simulink model "daohang_2017b"  (R2017b)
settings: Solver=FixedStepAuto  StartTime=0.0  StopTime=80  FixedStep=0.01  MaxStep=0.01  RelTol=1e-3
undefined symbols (not defined in the file or in its folder): Earth, ini, Newton, Raphson, WGS84
libraries: sharedutil x2, sharedtransform x2, simulink_extras x2, shared6dof x1, aerolibatmos2 x1, aerolibobsolete x1, aerolibtransform2 x1
(part 1 of 2)
settings Model: Creator=d8230  LastModifiedBy=d8230
settings SFSimCC: SimUseLocalCustomCode=on
settings RTWCC: RTWUseLocalCustomCode=on

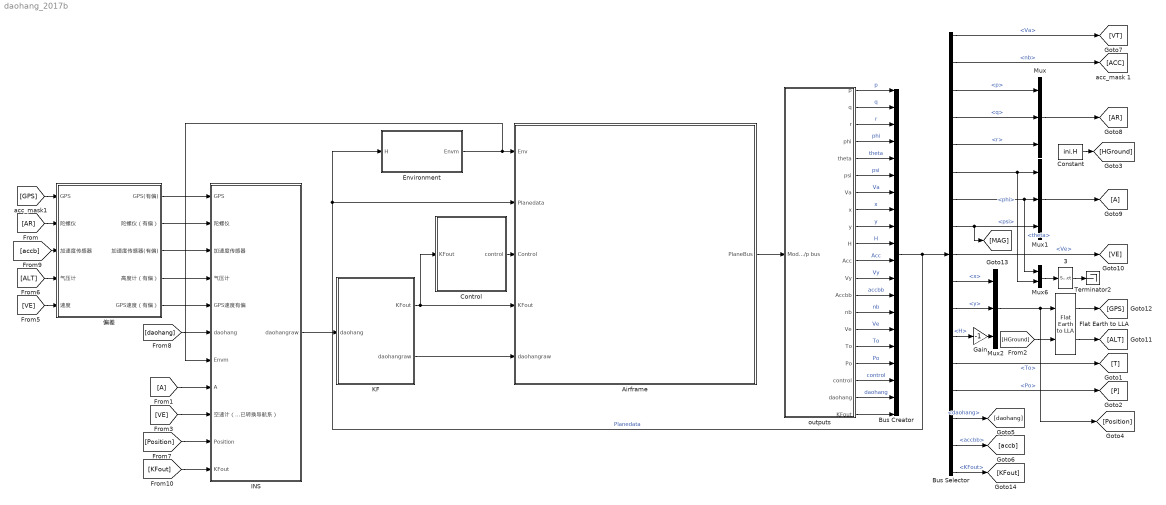
== system daohang_2017b ==
  3 : Selector  InputPortWidth=2  IndexOptions=Index vector (dialog)  Indices=[2,1]  OutputSizes=1
  Airframe : Subsystem
  Bus Creator : BusCreator  Inputs=20
  Bus Selector : BusSelector  OutputSignals=Va,nb,p,q,r,phi,theta,psi,Ve,x,y,H,To,Po,daohang,accbb,KFout
  Constant : Constant  Value=ini.H
  Control : Subsystem
  Environment : Subsystem  TreatAsAtomicUnit=on
  Flat Earth to LLA : aerolibtransform2/Flat Earth to LLA  units=Metric (MKS)  ptype=Earth (WGS84)  F=1/298.257223563  R=6378137  LL0=[30,100]  psi=0
  Gain : Gain  Gain=-1
  INS : Subsystem
  KF : Subsystem
  Mux : Mux  Inputs=3
  Mux1 : Mux  Inputs=3
  Mux2 : Mux  Inputs=3
  Mux6 : Mux  Inputs=2
  Terminator2 : Terminator
  outputs : Subsystem
  偏差 : Subsystem
  wires:
  Airframe/1(PlaneBus) -> outputs/1(Model o/p bus)
  Environment/1(Envm) -> INS/7(Envm), Airframe/1(Env)
  outputs/1(p) -> Bus Creator/1  "p"
  outputs/2(q) -> Bus Creator/2  "q"
  outputs/3(r) -> Bus Creator/3  "r"
  outputs/4(phi) -> Bus Creator/4  "phi"
  outputs/5(theta) -> Bus Creator/5  "theta"
  outputs/6(psi) -> Bus Creator/6  "psi"
  outputs/7(Va) -> Bus Creator/7  "Va"
  outputs/8(x) -> Bus Creator/8  "x"
  outputs/9(y) -> Bus Creator/9  "y"
  outputs/10(H) -> Bus Creator/10  "H"
  outputs/11(Acc) -> Bus Creator/11  "Acc"
  outputs/12(Vy) -> Bus Creator/12  "Vy"
  outputs/13(Accbb) -> Bus Creator/13  "accbb"
  outputs/15(Ve) -> Bus Creator/15  "Ve"
  outputs/14(nb) -> Bus Creator/14  "nb"
  Bus Creator/1 -> Environment/1(H), Airframe/2(Planedata), Bus Selector/1  "Planedata"
  Bus Selector/8 -> [MAG], Mux1/3  "<psi>"
  Mux6/1 -> 3/1
  Mux2/1 -> [Position], Flat Earth to LLA/1
  Bus Selector/10 -> Mux2/1  "<x>"
  Bus Selector/11 -> Mux2/2  "<y>"
  Gain/1 -> Mux2/3
  Bus Selector/13 -> [T]  "<To>"
  Bus Selector/14 -> [P]  "<Po>"
  Flat Earth to LLA/2 -> [ALT]
  Bus Selector/7 -> Mux6/1, Mux1/2  "<theta>"
  [HGround] -> Flat Earth to LLA/2
  Bus Selector/9 -> [VE]  "<Ve>"
  Bus Selector/5 -> Mux/3  "<r>"
  Bus Selector/12 -> Gain/1  "<H>"
  Flat Earth to LLA/1 -> [GPS]
  Bus Selector/1 -> [VT]  "<Va>"
  Mux/1 -> [AR]
  Bus Selector/3 -> Mux/1  "<p>"
  Bus Selector/4 -> Mux/2  "<q>"
  Bus Selector/2 -> [ACC]  "<nb>"
  Mux1/1 -> [A]
  3/1 -> Terminator2/1
  outputs/16(To) -> Bus Creator/16  "To"
  outputs/17(Po) -> Bus Creator/17  "Po"
  偏差/1(GPS(有偏)) -> INS/1(GPS)
  Constant/1 -> [HGround]
  [GPS] -> 偏差/1(GPS)
  [AR] -> 偏差/2(陀螺仪)
  INS/1(daohangraw) -> KF/1(daohang)
  Control/1(control) -> Airframe/3(Control)
  outputs/18(control) -> Bus Creator/18  "control"
  outputs/19(daohang) -> Bus Creator/19  "daohang"
  Bus Selector/15 -> [daohang]  "<daohang>"
  Bus Selector/16 -> [accb]  "<accbb>"
  [accb] -> 偏差/3(加速度传感器)
  [ALT] -> 偏差/4(气压计)
  KF/1(KFout) -> Control/1(KFout), Airframe/4(KFout)
  KF/2(daohangraw) -> Airframe/5(daohangraw)
  [daohang] -> INS/6(daohang)
  [A] -> INS/8(A)
  [VE] -> INS/9(空速计（已转换导航系）)
  [Position] -> INS/10(Position)
  偏差/2(陀螺仪（有偏）) -> INS/2(陀螺仪)
  偏差/3(加速度传感器(有偏)) -> INS/3(加速度传感器)
  偏差/4(高度计（有偏）) -> INS/4(气压计)
  Bus Selector/6 -> Mux6/2, Mux1/1  "<phi>"
  outputs/20("KFout ") -> Bus Creator/20
  [VE] -> 偏差/5(速度)
  偏差/5(GPS速度（有偏）) -> INS/5(GPS速度有偏)
  Bus Selector/17 -> [KFout]  "<KFout>"
  [KFout] -> INS/11("KFout ")

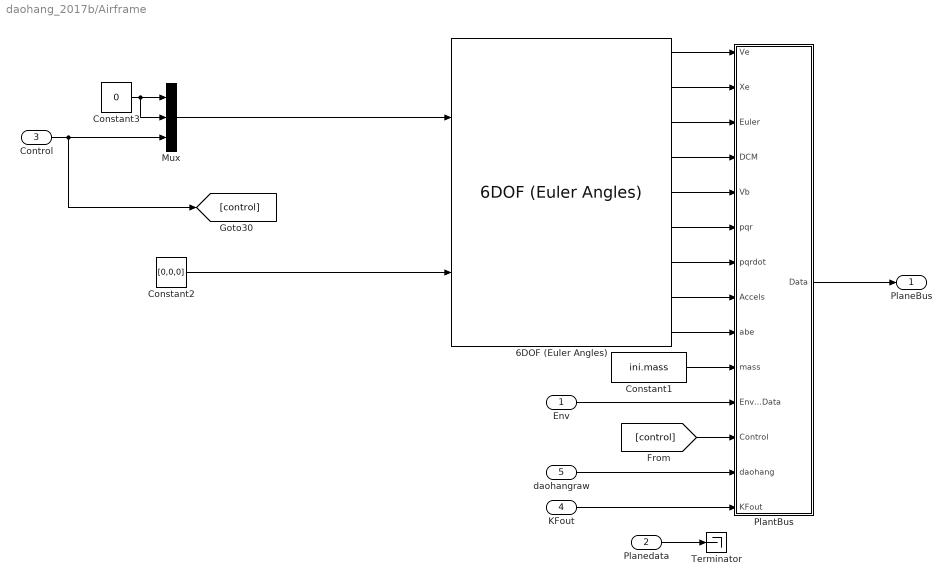
== system daohang_2017b/Airframe ==
  Env : Inport
  Planedata : Inport  Port=2
  Control : Inport  Port=3
  KFout : Inport  Port=4
  daohangraw : Inport  Port=5
  6DOF (Euler Angles) : shared6dof/6DOF (Euler Angles)  units=Metric (MKS)  mtype=Fixed  rep=Euler Angles  xme_0=ini.position  Vm_0=ini.Vb  eul_0=[ini.Euler(3),ini.Euler(2),ini.Euler(1)]  pm_0=ini.AR  mass_0=ini.mass  mass_e=0.5  mass_f=2.0  inertia=ini.inertia  inertia_e=eye(3)  inertia_f=2*eye(3)  k_quat=1.0  vre_flag=on  abi_flag=on
      settings: SourceProductBaseCode=AE
  Constant1 : Constant  Value=ini.mass
  Constant2 : Constant  Value=[0,0,0]
  Constant3 : Constant  Value=0
  Mux : Mux  Inputs=3
  PlantBus : Subsystem
  Terminator : Terminator
  PlaneBus : Outport
  wires:
  6DOF (Euler Angles)/1 -> PlantBus/1(Ve)
  6DOF (Euler Angles)/2 -> PlantBus/2(Xe)
  Mux/1 -> 6DOF (Euler Angles)/1
  6DOF (Euler Angles)/6 -> PlantBus/6(pqr)
  6DOF (Euler Angles)/4 -> PlantBus/4(DCM)
  6DOF (Euler Angles)/5 -> PlantBus/5(Vb)
  6DOF (Euler Angles)/8 -> PlantBus/8(Accels)
  6DOF (Euler Angles)/7 -> PlantBus/7(pqrdot)
  6DOF (Euler Angles)/3 -> PlantBus/3(Euler)
  6DOF (Euler Angles)/9 -> PlantBus/9(abe)
  PlantBus/1(Data) -> PlaneBus/1
  Env/1 -> PlantBus/11(EnvmData)
  Constant1/1 -> PlantBus/10(mass)
  Planedata/1 -> Terminator/1
  daohangraw/1 -> PlantBus/13(daohang)
  Constant2/1 -> 6DOF (Euler Angles)/2
  KFout/1 -> PlantBus/14(KFout)
  [control] -> PlantBus/12(Control)
  Constant3/1 -> Mux/2, Mux/1
  Control/1 -> Mux/3, [control]

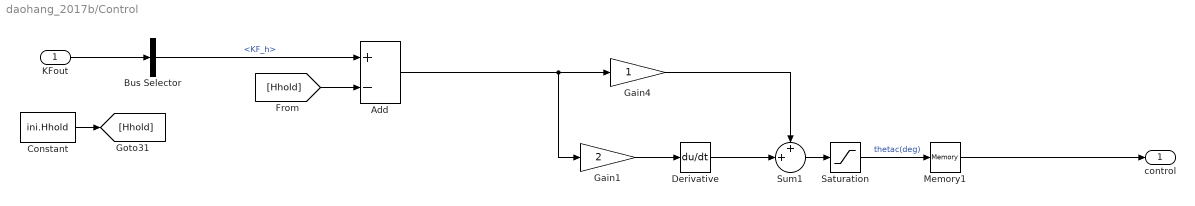
== system daohang_2017b/Control ==
  KFout : Inport
  Add : Sum  Inputs=+-
  Bus Selector : BusSelector  OutputSignals=KF_h
  Constant : Constant  Value=ini.Hhold
  Derivative : Derivative
  Gain1 : Gain  Gain=2
  Gain4 : Gain
  Memory1 : Memory
  Saturation : Saturate  UpperLimit=10  LowerLimit=-10
  Sum1 : Sum  Inputs=++|  SaturateOnIntegerOverflow=on
  control : Outport
  wires:
  KFout/1 -> Bus Selector/1
  Constant/1 -> [Hhold]
  [Hhold] -> Add/2
  Add/1 -> Gain1/1, Gain4/1
  Memory1/1 -> control/1
  Derivative/1 -> Sum1/2
  Sum1/1 -> Saturation/1
  Gain1/1 -> Derivative/1
  Saturation/1 -> Memory1/1  "thetac(deg)"
  Gain4/1 -> Sum1/1
  Bus Selector/1 -> Add/1  "<KF_h>"

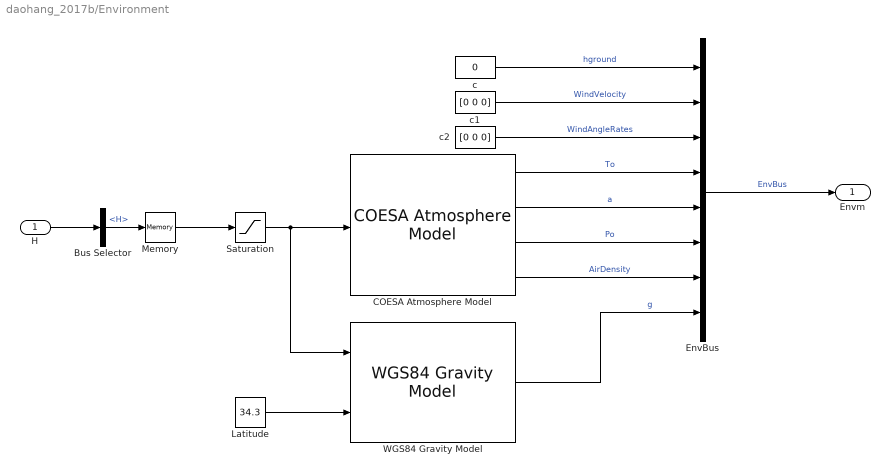
== system daohang_2017b/Environment ==
  H : Inport
  Bus Selector : BusSelector  OutputSignals=H
  COESA Atmosphere Model : aerolibatmos2/COESA Atmosphere Model  units=Metric (MKS)  spec=1976 COESA-extended U.S. Standard Atmosphere  model=Profile  profile_var=High temperature  profile_percent=1%  profile_alt=5 km (16404 ft)  envelope_var=High temperature  envelope_percent=1%  action=Warning
  EnvBus : BusCreator  Inputs=8
  Latitude : Constant  Value=34.3
  Memory : Memory  InitialCondition=-ini.position(3)
  Saturation : Saturate  UpperLimit=80000  LowerLimit=0
  WGS84 Gravity Model : aerolibobsolete/WGS84 Gravity Model  model=WGS84 Taylor Series  units=Metric (MKS)  no_atmos=on  precessing=on  month=February  day=1  year=2000  no_centrifugal=on  action=Warning
      settings: SourceProductName=Aerospace Blockset  SourceProductBaseCode=AE
  c : Constant  Value=0
  c1 : Constant  Value=[0 0 0]
  c2 : Constant  Value=[0 0 0]
  Envm : Outport
  wires:
  EnvBus/1 -> Envm/1  "EnvBus"
  Latitude/1 -> WGS84 Gravity Model/2
  H/1 -> Bus Selector/1
  Saturation/1 -> COESA Atmosphere Model/1, WGS84 Gravity Model/1
  c/1 -> EnvBus/1  "hground"
  c1/1 -> EnvBus/2  "WindVelocity"
  c2/1 -> EnvBus/3  "WindAngleRates"
  COESA Atmosphere Model/1 -> EnvBus/4  "To"
  COESA Atmosphere Model/2 -> EnvBus/5  "a"
  COESA Atmosphere Model/3 -> EnvBus/6  "Po"
  COESA Atmosphere Model/4 -> EnvBus/7  "AirDensity"
  WGS84 Gravity Model/1 -> EnvBus/8  "g"
  Memory/1 -> Saturation/1
  Bus Selector/1 -> Memory/1  "<H>"

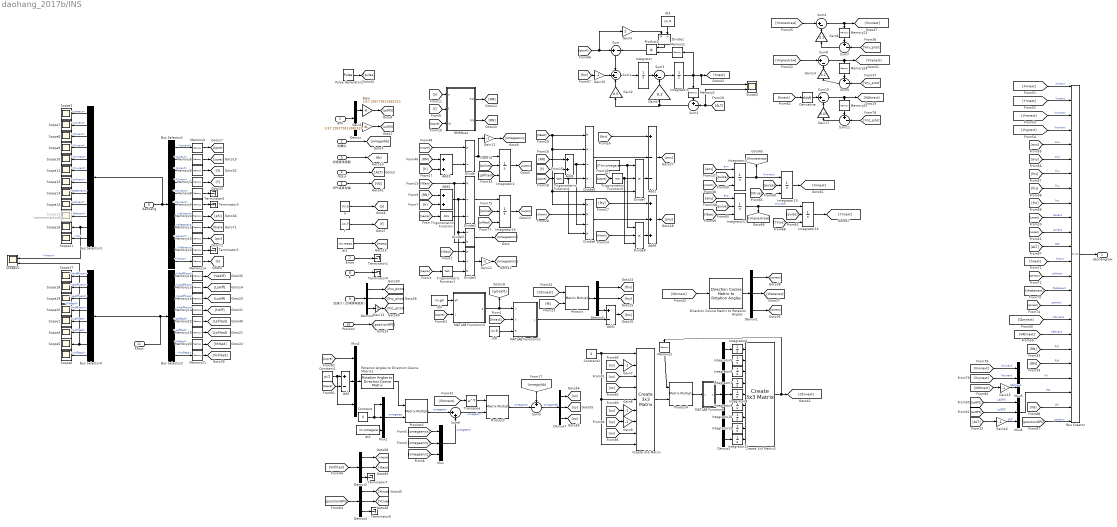
== system daohang_2017b/INS ==
  GPS : Inport
  陀螺仪 : Inport  Port=2
  加速度传感器 : Inport  Port=3
  气压计 : Inport  Port=4
  GPS速度有偏 : Inport  Port=5
  daohang : Inport  Port=6
  Envm : Inport  Port=7
  A : Inport  Port=8
  空速计（已转换导航系） : Inport  Port=9
  Position : Inport  Port=10
  "KFout " : Inport  Port=11
  Add : Sum  Inputs=+-
  Add1 : Sum  Inputs=+-
  Add2 : Sum  Inputs=+--
  Add3 : Sum
  Add4 : Sum
  Add5 : Sum
  Add6 : Sum  Inputs=+++
  Bus Creator : BusCreator  Inputs=24
  Bus Selector1 : BusSelector  OutputSignals=Lanext,Lonext,Xnnext,Ynnext,Vnxnext,Vnynext,phinext,thetanext,psinext,Valtnext,hnext
  Bus Selector2 : BusSelector  OutputSignals=Vediffnext,Ladiffnext,Lodiffnext,hdiffnext,Lafilted,Lofilted,hfilted,Vnfilted
  Bus Selector3 : BusSelector  OutputSignals=Lanext,Lonext,Xnnext,Ynnext,Vnxnext,Vnynext,phinext,thetanext,psinext,Valtnext,hnext,Vn
  Bus Selector4 : BusSelector  OutputSignals=Vediffnext,Ladiffnext,Lodiffnext,hdiffnext,Lafilted,Lofilted,hfilted,Vnfilted
  Constant : Constant  Value=0
  Constant1 : Constant  Value=pi/2
  Constant2 : Constant  Value=0
  Create 3x3 Matrix : sharedutil/Create 3x3 Matrix
  Create 3x3 Matrix1 : sharedutil/Create 3x3 Matrix
  Demux : Demux  Outputs=2
  Demux{1..5,7} (6 alike) : Demux  Outputs=3
  Demux9 : Demux  Outputs=9
  Derivative : Derivative
  Direction Cosine Matrix to Rotation Angles : sharedtransform/Direction Cosine Matrix to Rotation Angles  rotationOrder=ZYX
      settings: SourceProductName=Aerospace Blockset  SourceProductBaseCode=AE
  Divide : Product  Inputs=*/
  Divide1 : Product  Inputs=*/
  Divide2 : Product  Inputs=*//
  Divide3 : Product  Inputs=/*
  Divide4 : Product  Inputs=*/*
  Divide5 : Product  Inputs=**/*
  Divide6 : Product  Inputs=**/*
  Divide7 : Product  Inputs=***
  Divide8 : Product  Inputs=***
  Gain : Gain  Gain=1/57.295779513082323
  Gain1 : Gain  Gain=1/57.295779513082323
  Gain{7..13,15..16} (9 alike) : Gain  Gain=-1
  Gain14 : Gain  Gain=0.2
  Gain17 : Gain  Gain=0.01
  Gain2 : Gain  Gain=0.5
  Gain3 : Gain  Gain=2
  Gain4 : Gain  Gain=0.2
  Gain6 : Gain  Gain=0.2
  Integrator : Integrator  InitialCondition=-ini.Ve(3)
  Integrator1 : Integrator  InitialCondition=-ini.position(3)
  Integrator10 : Integrator  InitialCondition=ini.Cbn0(3,1)
  Integrator11 : Integrator  InitialCondition=ini.Cbn0(3,2)
  Integrator12 : Integrator  InitialCondition=ini.Cbn0(3,3)
  Integrator13 : Integrator  ExternalReset=rising  InitialConditionSource=external  InitialCondition=ini.position(1)
  Integrator14 : Integrator  ExternalReset=rising  InitialConditionSource=external  InitialCondition=ini.position(2)
  Integrator16 : Integrator  ExternalReset=rising  InitialConditionSource=external  InitialCondition=ini.Lo0/180*pi
  Integrator17 : Integrator  ExternalReset=rising  InitialConditionSource=external  InitialCondition=ini.Ve(1)
  Integrator2 : Integrator  ExternalReset=rising  InitialConditionSource=external  InitialCondition=ini.La0/180*pi
  Integrator3 : Integrator  ExternalReset=rising  InitialConditionSource=external  InitialCondition=ini.Ve(1)
  Integrator4 : Integrator  InitialCondition=ini.Cbn0(1,1)
  Integrator5 : Integrator  InitialCondition=ini.Cbn0(1,2)
  Integrator6 : Integrator  InitialCondition=ini.Cbn0(1,3)
  Integrator7 : Integrator  InitialCondition=ini.Cbn0(2,1)
  Integrator8 : Integrator  InitialCondition=ini.Cbn0(2,2)
  Integrator9 : Integrator
  MATLAB Function10 : MATLAB Function  TreatAsAtomicUnit=on
  MATLAB Function11 : MATLAB Function  TreatAsAtomicUnit=on
  MATLAB Function6 : MATLAB Function  TreatAsAtomicUnit=on
  Memory1 : Memory  InitialCondition=-ini.position(3)
  Memory10 : Memory  InitialCondition=ini.Euler(3)
  Memory11 : Memory  InitialCondition=ini.Euler(2)
  Memory12 : Memory  InitialCondition=ini.Euler(1)
  Memory13 : Memory  InitialCondition=ini.iniVe(3)
  Memory14 : Memory  InitialCondition=ini.iniH
  Memory15 : Memory  InitialCondition=ini.Ladiff
  Memory16 : Memory  InitialCondition=ini.Lodiff
  Memory17 : Memory  InitialCondition=ini.hdiff
  Memory18 : Memory  InitialCondition=ini.Vediff
  Memory19 : Memory  InitialCondition=ini.Lo0/180*pi
  Memory2 : Memory  InitialCondition=-ini.position(3)
  Memory20 : Memory  InitialCondition=-ini.position(3)
  Memory21 : Memory  InitialCondition=ini.Ve
  Memory22 : Memory  InitialCondition=ini.La0/180*pi
  Memory23 : Memory  InitialCondition=ini.Ve(1)
  Memory24 : Memory  InitialCondition=ini.Ve(2)
  Memory25 : Memory  InitialCondition=-ini.Ve(3)
  Memory3 : Memory  InitialCondition=ini.Cbn0
  Memory4 : Memory  InitialCondition=ini.iniLa/180*pi
  Memory5 : Memory  InitialCondition=ini.iniLo/180*pi
  Memory6 : Memory  InitialCondition=ini.position(1)
  Memory7 : Memory  InitialCondition=ini.position(1)
  Memory8 : Memory  InitialCondition=ini.Ve(1)
  Memory9 : Memory  InitialCondition=ini.Ve(2)
  Mux{,1..2,5..6} (5 alike) : Mux  Inputs=3
  Product{,2..4} (4 alike) : Product  Multiplication=Matrix(*)
  Product1 : Product
  Pulse Generator1 : DiscretePulseGenerator  Amplitude=10  Period=10000  PulseWidth=5  PhaseDelay=100  SampleTime=0.01
  RMRNcac : Subsystem
  Rotation Angles to Direction Cosine Matrix1 : sharedtransform/Rotation Angles to Direction Cosine Matrix  rotationOrder=ZYX
      settings: SourceProductBaseCode=AE
  Scope{1,3..14,16..21} (19 alike) : Scope
  Scope15 : Scope  Commented=on
  Scope2 : Scope  NumInputPorts=2
  Scope22 : Scope  NumInputPorts=2
  Sum : Sum  Inputs=+-
  Sum1 : Sum  Inputs=-+-
  Sum{3..4,8,10} (4 alike) : Sum  Inputs=|+-
  Sum{2,5,7,9,11} (5 alike) : Sum  Inputs=+-|
  Sum6 : Sum  Inputs=|++
  Terminator{1..7} (7 alike) : Terminator
  Transpose : Math  Operator=transpose  SaturateOnIntegerOverflow=on
  Trigonometric Function : Trigonometry  Operator=cos
  Trigonometric Function1 : Trigonometry  Operator=tan
  Trigonometric Function2 : Trigonometry  Operator=tan
  Trigonometric Function3 : Trigonometry
  a : Constant  Value=ini.a
  dt1 : Constant  Value=ini.mass
  dt2 : Constant  Value=ini.omegaie
  dt3 : Constant  Value=ini.g0
  dt4 : Constant  Value=ini.R
  dt7 : Constant  Value=2*ini.omegaie
  dt8 : Constant  Value=ini.R
  f : Constant  Value=ini.f
  daohangraw : Outport
  wires:
  GPS/1 -> Demux/1
  Demux/1 -> Gain/1
  Demux/2 -> Gain1/1
  气压计/1 -> [ALT]
  a/1 -> [a]
  f/1 -> [f]
  Gain1/1 -> [LoGPS]
  daohang/1 -> Bus Selector3/1, Bus Selector1/1
  dt1/1 -> [mass]
  加速度传感器/1 -> [fb]
  [fb] -> Product/2
  Demux3/3 -> Add1/1
  Demux3/1 -> [fnx]
  Product/1 -> Demux3/1
  Demux3/2 -> [fny]
  Position/1 -> [positionGPS]
  [Xnnext] -> Bus Creator/1  "Xnnext"
  [Ynnext] -> Bus Creator/2  "Ynnext"
  [Vnxnext] -> Bus Creator/3  "Vnxnext"
  [Vnynext] -> Bus Creator/4  "Vnynext"
  [anx] -> Bus Creator/5  "anx"
  [any] -> Bus Creator/6  "any"
  [fnx] -> Bus Creator/7  "fnx"
  [fny] -> Bus Creator/8  "fny"
  [fnz] -> Bus Creator/9  "fnz"
  [Lanext] -> Bus Creator/10  "Lanext"
  [Lonext] -> Bus Creator/11  "Lonext"
  [Cbnnext] -> Product/1
  [Lapre] -> MATLAB Function10/2(L)
  Demux1/3 -> [phinext]
  Demux1/2 -> [thetanext]
  Demux1/1 -> [psinext]
  dt3/1 -> MATLAB Function10/1(g0)
  [glocal0] -> Gain3/1, Sum/1
  Gain3/1 -> Divide1/1
  dt4/1 -> Divide1/2
  Divide1/1 -> Product1/1
  Sum/1 -> Sum1/1
  Gain2/1 -> Sum1/3
  Sum2/1 -> Gain2/1, Gain4/1
  Sum1/1 -> Integrator/1
  Integrator/1 -> Sum3/1
  Gain4/1 -> Sum3/2
  Sum3/1 -> Integrator1/1
  Product1/1 -> Sum/2
  [hnext] -> Bus Creator/13  "hnext"
  [phinext] -> Bus Creator/14  "phinext"
  [thetanext] -> Bus Creator/15  "thetanext"
  [psinext] -> Bus Creator/16  "psinext"
  陀螺仪/1 -> [omegaibb]
  dt2/1 -> Mux1/3
  Constant/1 -> Mux1/1, Mux1/2
  Rotation Angles to Direction Cosine Matrix1/1 -> Product2/1
  Mux1/1 -> Product2/2  "omegaiee"
  Constant1/1 -> Mux2/3, Add/1
  Mux2/1 -> Rotation Angles to Direction Cosine Matrix1/1
  [Lopre] -> Mux2/1
  Add/1 -> Mux2/2
  [Lapre] -> Add/2
  Product2/1 -> Sum6/1  "omegaien"
  Mux/1 -> Sum6/2  "omegaenn"
  Sum6/1 -> Product3/2  "omegainn"
  [Cbnnext] -> Transpose/1
  Transpose/1 -> Product3/1
  Constant2/1 -> Create 3x3 Matrix/9, Create 3x3 Matrix/5, Create 3x3 Matrix/1
  Sum5/1 -> Demux7/1  "omeganbb"
  Demux7/2 -> [oy]
  Demux7/1 -> [ox]
  Demux7/3 -> [oz]
  [oz] -> Gain7/1
  Gain7/1 -> Create 3x3 Matrix/2
  [oy] -> Create 3x3 Matrix/3
  [oz] -> Create 3x3 Matrix/4
  [ox] -> Gain8/1
  Gain8/1 -> Create 3x3 Matrix/6
  [oy] -> Gain9/1
  Gain9/1 -> Create 3x3 Matrix/7
  [ox] -> Create 3x3 Matrix/8
  Create 3x3 Matrix/1 -> Product4/2
  [Cbnnext] -> Bus Creator/17  "Cbnnext"
  Product4/1 -> MATLAB Function6/1(u)
  Demux9/1 -> Integrator4/1
  Integrator4/1 -> Create 3x3 Matrix1/1
  Integrator5/1 -> Create 3x3 Matrix1/2
  Demux9/2 -> Integrator5/1
  Integrator6/1 -> Create 3x3 Matrix1/3
  Demux9/3 -> Integrator6/1
  Integrator7/1 -> Create 3x3 Matrix1/4
  Demux9/4 -> Integrator7/1
  Integrator8/1 -> Create 3x3 Matrix1/5
  Demux9/5 -> Integrator8/1
  Integrator9/1 -> Create 3x3 Matrix1/6
  Demux9/6 -> Integrator9/1
  Integrator10/1 -> Create 3x3 Matrix1/7
  Demux9/7 -> Integrator10/1
  Integrator11/1 -> Create 3x3 Matrix1/8
  Demux9/8 -> Integrator11/1
  Integrator12/1 -> Create 3x3 Matrix1/9
  Demux9/9 -> Integrator12/1
  Bus Creator/1 -> daohangraw/1
  [omegaibb] -> Sum5/1
  [ALT] -> Bus Creator/12  "ALT"
  [fnz] -> Gain10/1
  Integrator1/1 -> Memory2/1, Scope2/1, [hnext], Memory1/1
  Memory1/1 -> Product1/2
  Memory2/1 -> Sum2/1
  Add1/1 -> [fnz]
  MATLAB Function10/1(g) -> MATLAB Function11/1(u), [glocal0]
  [hnext] -> MATLAB Function11/2(h)
  dt8/1 -> MATLAB Function11/3(R)
  MATLAB Function11/1(y) -> Add1/2
  [ALT] -> Scope2/2, Sum2/2
  Gain10/1 -> Sum1/2
  Integrator13/1 -> [Xnnext]
  Integrator14/1 -> [Ynnext]
  Product3/1 -> Sum5/2  "omegainb"
  Bus Selector1/10 -> Memory13/1  "<Valtnext>"
  Bus Selector1/6 -> Memory9/1  "<Vnynext>"
  Bus Selector1/3 -> Memory6/1  "<Xnnext>"
  Bus Selector1/4 -> Memory7/1  "<Ynnext>"
  Bus Selector1/5 -> Memory8/1  "<Vnxnext>"
  Bus Selector1/9 -> Memory12/1  "<psinext>"
  Bus Selector1/8 -> Memory11/1  "<thetanext>"
  Bus Selector1/7 -> Memory10/1  "<phinext>"
  Memory6/1 -> [X]
  Memory7/1 -> [Y]
  Memory8/1 -> Terminator5/1
  Memory9/1 -> Terminator3/1
  Memory10/1 -> [phi]
  Memory11/1 -> [theta]
  Memory12/1 -> [psi]
  [hnext] -> Derivative/1
  [VAltnext] -> Bus Creator/18  "Valtnext"
  Memory13/1 -> Terminator2/1
  Envm/1 -> Terminator1/1
  A/1 -> Terminator4/1
  [RN] -> Bus Creator/19  "RN"
  [RM] -> Bus Creator/20  "RM"
  MATLAB Function6/1(y) -> Demux9/1
  Direction Cosine Matrix to Rotation Angles/1 -> Demux1/1
  [Cbnnext] -> Direction Cosine Matrix to Rotation Angles/1
  Bus Selector1/11 -> Memory14/1  "<hnext>"
  Memory14/1 -> [h]
  [RM] -> Add3/1
  [h] -> Add3/2
  [VNorth] -> Divide/1
  Add3/1 -> Divide/2
  Divide/1 -> Gain11/1, Integrator2/1
  [Lapre] -> Trigonometric Function/1
  Trigonometric Function/1 -> Divide2/3
  [RN] -> Add4/1
  [h] -> Add4/2
  Add4/1 -> Divide4/2, Divide3/1, Divide2/2
  [VEast] -> Divide3/2, Divide2/1
  Divide2/1 -> Integrator16/1
  [a] -> RMRNcac/1(a)
  [f] -> RMRNcac/2(f)
  [Lapre] -> RMRNcac/3(La)
  RMRNcac/1(RM) -> [RM]
  RMRNcac/2(RN) -> [RN]
  Divide3/1 -> [omegaennx]
  Gain11/1 -> [omegaenny]
  [VEast] -> Divide4/1
  [Lapre] -> Trigonometric Function1/1
  Trigonometric Function1/1 -> Divide4/3
  Divide4/1 -> Gain12/1
  Gain12/1 -> [omegaennz]
  [omegaennx] -> Mux/1
  [omegaenny] -> Mux/2
  [omegaennz] -> Mux/3
  Gain/1 -> [LaGPS]
  Memory4/1 -> [Lapre]
  Memory5/1 -> [Lopre]
  Bus Selector1/2 -> Memory5/1  "<Lonext>"
  Bus Selector1/1 -> Memory4/1  "<Lanext>"
  [fnx] -> Add2/1
  [h] -> Add5/2
  [RN] -> Add5/1
  Add5/1 -> Divide5/3, Divide6/3
  [Lapre] -> Trigonometric Function2/1
  Trigonometric Function2/1 -> Divide5/4, Divide6/4
  Divide5/1 -> Add2/2
  Add2/1 -> [anx]
  [fny] -> Add6/1
  Add6/1 -> [any]
  Divide6/1 -> Add6/2
  dt7/1 -> Divide7/1, Divide8/1
  [Lapre] -> Trigonometric Function3/1
  Divide7/1 -> Add2/3
  [VNorth] -> Divide6/2
  [VEast] -> Divide5/1, Divide5/2, Divide7/3, Divide6/1
  Divide8/1 -> Add6/3
  [VNorth] -> Divide8/2
  Trigonometric Function3/1 -> Divide7/2, Divide8/3
  Integrator2/1 -> [Lanext]
  Integrator16/1 -> [Lonext]
  Bus Selector2/1 -> Memory18/1  "<Vediffnext>"
  Bus Selector2/2 -> Memory15/1  "<Ladiffnext>"
  Bus Selector2/3 -> Memory16/1  "<Lodiffnext>"
  Bus Selector2/4 -> Memory17/1  "<hdiffnext>"
  Integrator3/1 -> [Vnxnextraw], Integrator13/1  "Vnxnext"
  Integrator17/1 -> [Vnynextraw], Integrator14/1  "Vnynext"
  [anx] -> Integrator3/1  "anx"
  [any] -> Integrator17/1  "any"
  [VAltnext] -> Gain15/1
  [Vnxnext] -> Mux5/1  "Vnxnext"
  [Vnynext] -> Mux5/2  "Vnynext"
  Gain15/1 -> Mux5/3  "VAltnext-"
  Mux5/1 -> Bus Creator/21  "Vn"
  [LoGPS] -> Mux6/2  "LoGPS"
  Gain16/1 -> Mux6/3  "ALT"
  [ALT] -> Gain16/1
  [LaGPS] -> Mux6/1  "LaGPS"
  Mux6/1 -> Bus Creator/22  "PG"
  [VG] -> Bus Creator/23  "VG"
  [positionGPS] -> Bus Creator/24  "position"
  GPS速度有偏/1 -> [VG]
  Memory18/1 -> [Vediff]
  Memory15/1 -> [Ladiff]
  Memory17/1 -> [hdiff]
  Memory16/1 -> [Lodiff]
  Bus Selector3/10 -> Scope15/1  "<Valtnext>"
  Bus Selector3/1 -> Scope3/1  "<Lanext>"
  Bus Selector3/5 -> Scope10/1  "<Vnxnext>"
  Bus Selector3/11 -> Scope22/1, Scope16/1  "<hnext>"
  Bus Selector3/7 -> Scope12/1  "<phinext>"
  Bus Selector3/8 -> Scope13/1  "<thetanext>"
  Bus Selector4/1 -> Scope17/1  "<Vediffnext>"
  Bus Selector4/2 -> Scope18/1  "<Ladiffnext>"
  Bus Selector4/3 -> Scope19/1  "<Lodiffnext>"
  Bus Selector3/9 -> Scope14/1  "<psinext>"
  Bus Selector3/6 -> Scope11/1  "<Vnynext>"
  "KFout "/1 -> Bus Selector4/1, Bus Selector2/1
  Bus Selector3/2 -> Scope7/1  "<Lonext>"
  Bus Selector4/4 -> Scope20/1  "<hdiffnext>"
  Bus Selector3/4 -> Scope9/1  "<Ynnext>"
  Bus Selector3/3 -> Scope8/1  "<Xnnext>"
  Memory3/1 -> Product4/1
  Bus Selector2/7 -> Memory20/1  "<hfilted>"
  Memory21/1 -> [Vnfilted]
  Memory19/1 -> [Lofilted]
  Bus Selector2/5 -> Memory22/1  "<Lafilted>"
  Memory22/1 -> [Lafilted]
  Memory20/1 -> [hfilted]
  Bus Selector2/6 -> Memory19/1  "<Lofilted>"
  Bus Selector2/8 -> Memory21/1  "<Vnfilted>"
  Bus Selector4/5 -> Scope1/1  "<Lafilted>"
  Bus Selector4/6 -> Scope4/1  "<Lofilted>"
  Bus Selector4/7 -> Scope5/1, Scope22/2  "<hfilted>"
  Bus Selector4/8 -> Scope6/1  "<Vnfilted>"
  Bus Selector3/12 -> Scope21/1  "<Vn>"
  Create 3x3 Matrix1/1 -> [Cbnnext], Memory3/1
  [pulse] -> Integrator2/2
  [Lafilted] -> Integrator2/3
  [pulse] -> Integrator3/2
  [Vnfilted] -> Demux2/1
  Demux2/1 -> [VNorth]
  Demux2/2 -> [VEast]
  Demux2/3 -> Terminator7/1
  [VNorth] -> Integrator3/3
  [pulse] -> Integrator17/2
  [VEast] -> Integrator17/3
  [pulse] -> Integrator14/2
  Demux4/1 -> [Xtrue]
  [positionGPS] -> Demux4/1
  Demux4/3 -> Terminator6/1
  Demux4/2 -> [Ytrue]
  [Ytrue] -> Integrator14/3
  [Xtrue] -> Integrator13/3
  [pulse] -> Integrator13/2
  Pulse Generator1/1 -> [pulse]
  [pulse] -> Integrator16/2
  [Lofilted] -> Integrator16/3
  [Vnxnextraw] -> Sum4/1
  [Vnx_pitot] -> Sum7/2
  Sum7/1 -> Gain6/1
  Memory23/1 -> Sum7/1
  Gain6/1 -> Sum4/2
  Demux5/2 -> [Vny_pitot]
  空速计（已转换导航系）/1 -> Demux5/1
  Demux5/3 -> Gain13/1
  Demux5/1 -> [Vnx_pitot]
  Gain13/1 -> [Vnz_pitot]
  Sum4/1 -> [Vnxnext], Memory23/1
  Memory24/1 -> Sum9/1
  [Vny_pitot] -> Sum9/2
  [Vnynextraw] -> Sum8/1
  Sum8/1 -> [Vnynext], Memory24/1
  Gain14/1 -> Sum8/2
  Sum9/1 -> Gain14/1
  Memory25/1 -> Sum11/1
  [Vnz_pitot] -> Sum11/2
  Derivative/1 -> Sum10/1
  Sum10/1 -> [VAltnext], Memory25/1
  Gain17/1 -> Sum10/2
  Sum11/1 -> Gain17/1

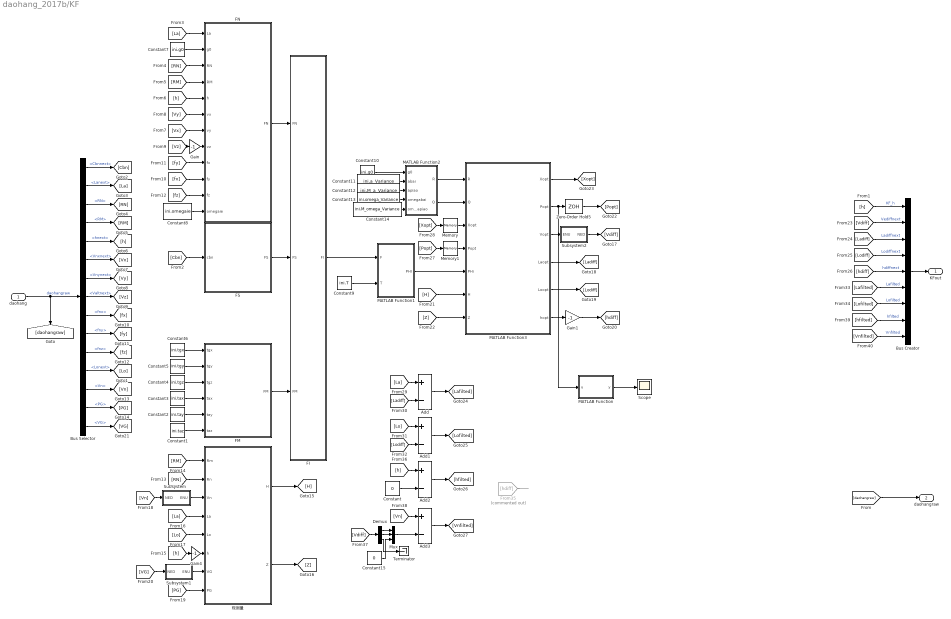
== system daohang_2017b/KF ==
  daohang : Inport
  Add{,1..3} (4 alike) : Sum  Inputs=+-
  Bus Creator : BusCreator  Inputs=9
  Bus Selector : BusSelector  OutputSignals=Cbnnext,Lanext,RN,RM,hnext,Vnxnext,Vnynext,Valtnext,fnx,fny,fnz,Lonext,Vn,PG,VG
  Constant : Constant  Value=0
  Constant1 : Constant  Value=ini.taz
  Constant10 : Constant  Value=ini.g0
  Constant11 : Constant  Value=ini.a_Variance
  Constant12 : Constant  Value=ini.M_a_Variance
  Constant13 : Constant  Value=ini.omega_Variance
  Constant14 : Constant  Value=ini.M_omega_Variance
  Constant15 : Constant  Value=0
  Constant2 : Constant  Value=ini.tay
  Constant3 : Constant  Value=ini.tax
  Constant4 : Constant  Value=ini.tgz
  Constant5 : Constant  Value=ini.tgy
  Constant6 : Constant  Value=ini.tgx
  Constant7 : Constant  Value=ini.g0
  Constant8 : Constant  Value=ini.omegaie
  Constant9 : Constant  Value=ini.T
  Demux : Demux  Outputs=3
  FI : MATLAB Function  TreatAsAtomicUnit=on
  FM : MATLAB Function  TreatAsAtomicUnit=on
  "FN " : MATLAB Function  TreatAsAtomicUnit=on
  FS : MATLAB Function  TreatAsAtomicUnit=on
  From35 : From  Commented=on  GotoTag=hdiff
  Gain : Gain  Gain=-1
  Gain1 : Gain  Gain=-1
  Gain4 : Gain  Gain=-1
  MATLAB Function : MATLAB Function  TreatAsAtomicUnit=on
  MATLAB Function1 : MATLAB Function  TreatAsAtomicUnit=on
  MATLAB Function2 : MATLAB Function  TreatAsAtomicUnit=on
  MATLAB Function3 : MATLAB Function  TreatAsAtomicUnit=on
  Memory : Memory  InitialCondition=ini.Xopt0
  Memory1 : Memory  InitialCondition=ini.Popt0
  Mux : Mux  Inputs=3
  Scope : Scope
  Subsystem : Subsystem
  Subsystem1 : Subsystem
  Subsystem2 : Subsystem
  Terminator : Terminator
  Zero-Order Hold5 : ZeroOrderHold
  观测量 : MATLAB Function  TreatAsAtomicUnit=on
  KFout : Outport
  daohangraw : Outport  Port=2
  wires:
  daohang/1 -> [daohangraw], Bus Selector/1  "daohangraw"
  Bus Creator/1 -> KFout/1
  [h] -> Bus Creator/1  "KF_h"
  Constant1/1 -> FM/6(taz)
  Constant2/1 -> FM/5(tay)
  Constant3/1 -> FM/4(tax)
  Constant5/1 -> FM/2(tgy)
  Constant4/1 -> FM/3(tgz)
  Constant6/1 -> FM/1(tgx)
  Bus Selector/1 -> [Cbn]  "<Cbnnext>"
  [Cbn] -> FS/1(cbn)
  Bus Selector/2 -> [La]  "<Lanext>"
  Bus Selector/3 -> [RN]  "<RN>"
  Bus Selector/4 -> [RM]  "<RM>"
  Bus Selector/5 -> [h]  "<hnext>"
  Bus Selector/6 -> [Vx]  "<Vnxnext>"
  Bus Selector/7 -> [Vy]  "<Vnynext>"
  Bus Selector/8 -> [Vz]  "<Valtnext>"
  Bus Selector/9 -> [fx]  "<fnx>"
  Bus Selector/10 -> [fy]  "<fny>"
  Bus Selector/11 -> [fz]  "<fnz>"
  [La] -> "FN "/1(La)
  Constant7/1 -> "FN "/2(g0)
  [RN] -> "FN "/3(RN)
  [RM] -> "FN "/4(RM)
  [h] -> "FN "/5(h)
  [Vx] -> "FN "/7(vy)
  [Vy] -> "FN "/6(vx)
  [Vz] -> Gain/1
  Gain/1 -> "FN "/8(vz)
  [fx] -> "FN "/10(fy)
  [fy] -> "FN "/9(fx)
  [fz] -> "FN "/11(fz)
  Constant8/1 -> "FN "/12(omegaie)
  "FN "/1(FN) -> FI/1(FN)
  FS/1(FS) -> FI/2(FS)
  FM/1(FM) -> FI/3(FM)
  FI/1(FI) -> MATLAB Function1/1(F)
  Constant9/1 -> MATLAB Function1/2(T)
  [RM] -> 观测量/1(Rm)
  [RN] -> 观测量/2(Rn)
  [h] -> Gain4/1
  [La] -> 观测量/4(La)
  Bus Selector/12 -> [Lo]  "<Lonext>"
  [Lo] -> 观测量/5(Lo)
  Bus Selector/13 -> [Vn]  "<Vn>"
  Bus Selector/14 -> [PG]  "<PG>"
  [PG] -> 观测量/8(PG)
  [VG] -> Subsystem1/1("NED ")
  观测量/1(H) -> [H]
  观测量/2(Z) -> [Z]
  Constant10/1 -> MATLAB Function2/1(g0)
  Constant11/1 -> MATLAB Function2/2(abai)
  Constant12/1 -> MATLAB Function2/3(apiao)
  Constant13/1 -> MATLAB Function2/4(omegabai)
  Constant14/1 -> MATLAB Function2/5(omegapiao)
  Gain1/1 -> [hdiff]
  [Vdiff] -> Bus Creator/2  "Vediffnext"
  [Ladiff] -> Bus Creator/3  "Ladiffnext"
  [Lodiff] -> Bus Creator/4  "Lodiffnext"
  [hdiff] -> Bus Creator/5  "hdiffnext"
  [daohangraw] -> daohangraw/1
  Gain4/1 -> 观测量/6(h)
  Bus Selector/15 -> [VG]  "<VG>"
  [Vn] -> Subsystem/1("NED ")
  Subsystem/1(ENU) -> 观测量/3(Vn)
  Subsystem1/1(ENU) -> 观测量/7(VG)
  Subsystem2/1(NED) -> [Vdiff]
  [Popt] -> Memory1/1
  [Xopt] -> Memory/1
  [La] -> Add/1
  [Ladiff] -> Add/2
  Add/1 -> [Lafilted]
  [Lo] -> Add1/1
  [Lodiff] -> Add1/2
  Add1/1 -> [Lofilted]
  [h] -> Add2/1
  From35/1 -> ?
  Add2/1 -> [hfilted]
  [Vn] -> Add3/1
  [Vdiff] -> Demux/1
  Add3/1 -> [Vnfilted]
  [Lafilted] -> Bus Creator/6  "Lafilted"
  [Lofilted] -> Bus Creator/7  "Lofilted"
  [hfilted] -> Bus Creator/8  "hfilted"
  [Vnfilted] -> Bus Creator/9  "Vnfilted"
  Zero-Order Hold5/1 -> [Popt]
  MATLAB Function/1(y) -> Scope/1
  Memory/1 -> MATLAB Function3/3("Xopt ")
  Memory1/1 -> MATLAB Function3/4("Popt ")
  MATLAB Function2/2(Q) -> MATLAB Function3/2(Q)
  MATLAB Function2/1(R) -> MATLAB Function3/1(R)
  MATLAB Function1/1(PHI) -> MATLAB Function3/5(PHi)
  [H] -> MATLAB Function3/6(H)
  [Z] -> MATLAB Function3/7(Z)
  MATLAB Function3/1(Xopt) -> [Xopt]
  MATLAB Function3/2(Popt) -> MATLAB Function/1(u), Zero-Order Hold5/1
  MATLAB Function3/3(Vopt) -> Subsystem2/1("ENU ")
  MATLAB Function3/4(Laopt) -> [Ladiff]
  MATLAB Function3/5(Loopt) -> [Lodiff]
  MATLAB Function3/6(hopt) -> Gain1/1
  Constant/1 -> Add2/2
  Demux/1 -> Mux/1
  Demux/2 -> Mux/2
  Constant15/1 -> Mux/3
  Mux/1 -> Add3/2
  Demux/3 -> Terminator/1

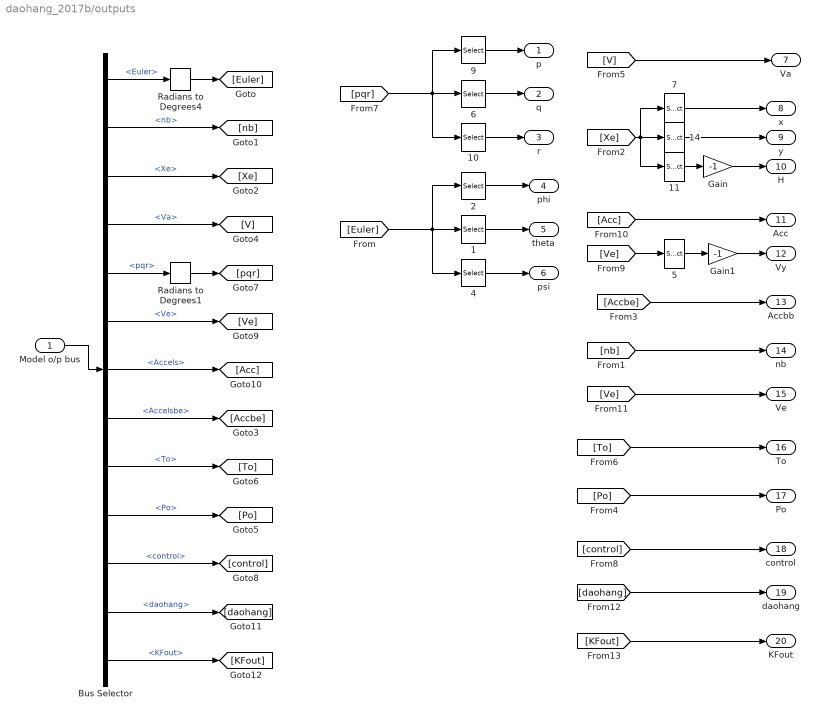
== system daohang_2017b/outputs ==
  Model o/p bus : Inport
  {1,5..6,14} (4 alike) : Selector  InputPortWidth=3  IndexOptions=Index vector (dialog)  Indices=2  OutputSizes=1
  10 : Selector  InputPortWidth=3  IndexOptions=Index vector (dialog)  Indices=3  OutputSizes=1
  11 : Selector  InputPortWidth=3  IndexOptions=Index vector (dialog)  Indices=3  OutputSizes=1
  2 : Selector  InputPortWidth=3  IndexOptions=Index vector (dialog)  Indices=1  OutputSizes=1
  4 : Selector  InputPortWidth=3  IndexOptions=Index vector (dialog)  Indices=3  OutputSizes=1
  7 : Selector  InputPortWidth=3  IndexOptions=Index vector (dialog)  Indices=1  OutputSizes=1
  9 : Selector  InputPortWidth=3  IndexOptions=Index vector (dialog)  Indices=1  OutputSizes=1
  Bus Selector : BusSelector  OutputSignals=Euler,nb,Xe,Va,pqr,Ve,Accels,Accelsbe,To,Po,control,daohang,KFout
  Gain : Gain  Gain=-1
  Gain1 : Gain  Gain=-1
  Radians to Degrees1 : simulink_extras/Transformations/Radians to Degrees
  Radians to Degrees4 : simulink_extras/Transformations/Radians to Degrees
  p : Outport
  q : Outport  Port=2
  r : Outport  Port=3
  phi : Outport  Port=4
  theta : Outport  Port=5
  psi : Outport  Port=6
  Va : Outport  Port=7
  x : Outport  Port=8
  y : Outport  Port=9
  H : Outport  Port=10
  Acc : Outport  Port=11
  Vy : Outport  Port=12
  Accbb : Outport  Port=13
  nb : Outport  Port=14
  Ve : Outport  Port=15
  To : Outport  Port=16
  Po : Outport  Port=17
  control : Outport  Port=18
  daohang : Outport  Port=19
  "KFout " : Outport  Port=20
  wires:
  Bus Selector/5 -> Radians to Degrees1/1  "<pqr>"
  Bus Selector/4 -> [V]  "<Va>"
  Bus Selector/2 -> [nb]  "<nb>"
  Bus Selector/1 -> Radians to Degrees4/1  "<Euler>"
  Bus Selector/3 -> [Xe]  "<Xe>"
  Model o/p bus/1 -> Bus Selector/1
  Bus Selector/6 -> [Ve]  "<Ve>"
  6/1 -> q/1
  9/1 -> p/1
  [pqr] -> 6/1, 9/1, 10/1
  10/1 -> r/1
  [Euler] -> 4/1, 1/1, 2/1
  4/1 -> psi/1
  2/1 -> phi/1
  1/1 -> theta/1
  14/1 -> y/1
  Gain/1 -> H/1
  11/1 -> Gain/1
  [Xe] -> 11/1, 14/1, 7/1
  Gain1/1 -> Vy/1
  5/1 -> Gain1/1
  [Ve] -> 5/1
  7/1 -> x/1
  [V] -> Va/1
  Radians to Degrees1/1 -> [pqr]
  Radians to Degrees4/1 -> [Euler]
  [nb] -> nb/1
  Bus Selector/7 -> [Acc]  "<Accels>"
  [Acc] -> Acc/1
  [Ve] -> Ve/1
  Bus Selector/8 -> [Accbe]  "<Accelsbe>"
  [Accbe] -> Accbb/1
  Bus Selector/9 -> [To]  "<To>"
  Bus Selector/10 -> [Po]  "<Po>"
  [Po] -> Po/1
  [To] -> To/1
  Bus Selector/11 -> [control]  "<control>"
  Bus Selector/12 -> [daohang]  "<daohang>"
  [control] -> control/1
  [daohang] -> daohang/1
  Bus Selector/13 -> [KFout]  "<KFout>"
  [KFout] -> "KFout "/1

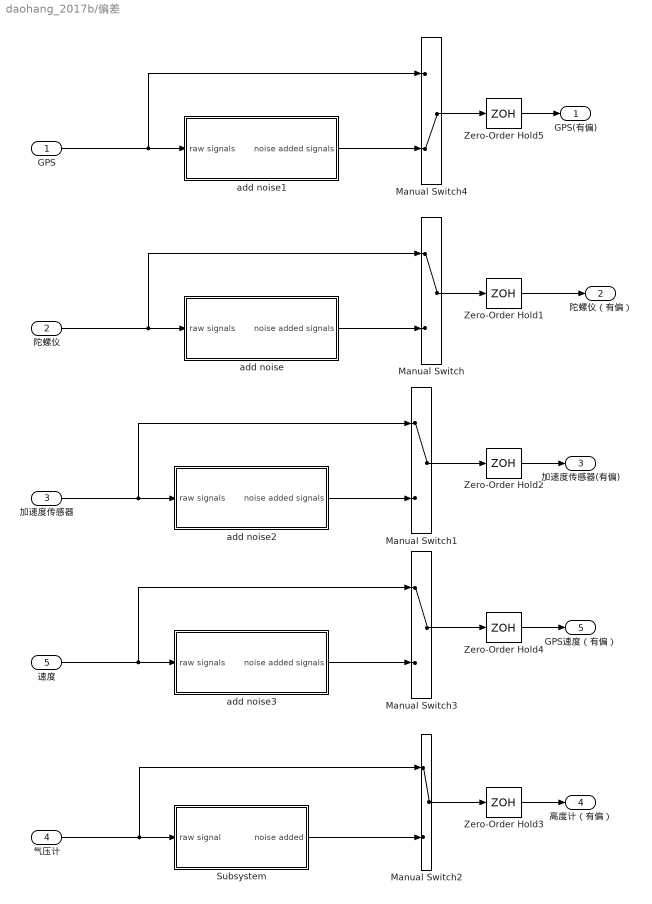
== system daohang_2017b/偏差 ==
  GPS : Inport
  陀螺仪 : Inport  Port=2
  加速度传感器 : Inport  Port=3
  气压计 : Inport  Port=4
  速度 : Inport  Port=5
  Manual Switch{,1..3} (4 alike) : ManualSwitch
  Manual Switch4 : ManualSwitch  CurrentSetting=0
  Subsystem : Subsystem
  Zero-Order Hold{1..5} (5 alike) : ZeroOrderHold  SampleTime=0.01
  add noise : Subsystem
  add noise1 : Subsystem
  add noise2 : Subsystem
  add noise3 : Subsystem
  GPS(有偏) : Outport
  陀螺仪（有偏） : Outport  Port=2
  加速度传感器(有偏) : Outport  Port=3
  高度计（有偏） : Outport  Port=4
  GPS速度（有偏） : Outport  Port=5
  wires:
  陀螺仪/1 -> add noise/1(raw signals), Manual Switch/1
  气压计/1 -> Subsystem/1(raw signal), Manual Switch2/1
  Manual Switch/1 -> Zero-Order Hold1/1
  Manual Switch2/1 -> Zero-Order Hold3/1
  Zero-Order Hold1/1 -> 陀螺仪（有偏）/1
  Zero-Order Hold2/1 -> 加速度传感器(有偏)/1
  Zero-Order Hold3/1 -> 高度计（有偏）/1
  Zero-Order Hold4/1 -> GPS速度（有偏）/1
  Zero-Order Hold5/1 -> GPS(有偏)/1
  add noise/1(noise added signals) -> Manual Switch/2
  Manual Switch4/1 -> Zero-Order Hold5/1
  GPS/1 -> add noise1/1(raw signals), Manual Switch4/1
  add noise1/1(noise added signals) -> Manual Switch4/2
  Manual Switch1/1 -> Zero-Order Hold2/1
  加速度传感器/1 -> add noise2/1(raw signals), Manual Switch1/1
  add noise2/1(noise added signals) -> Manual Switch1/2
  Manual Switch3/1 -> Zero-Order Hold4/1
  速度/1 -> add noise3/1(raw signals), Manual Switch3/1
  add noise3/1(noise added signals) -> Manual Switch3/2
  Subsystem/1(noise added) -> Manual Switch2/2

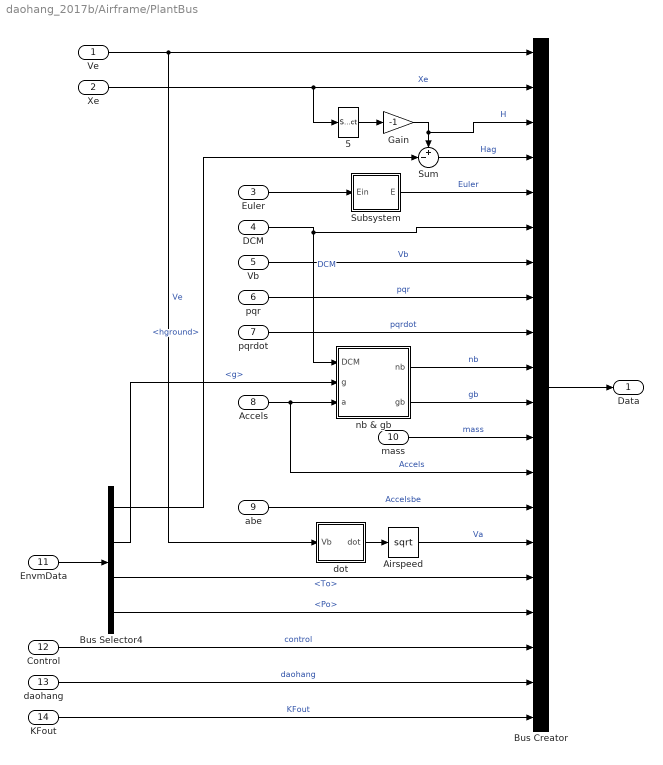
== system daohang_2017b/Airframe/PlantBus ==
  Ve : Inport
  Xe : Inport  Port=2
  Euler : Inport  Port=3
  DCM : Inport  Port=4
  Vb : Inport  Port=5
  pqr : Inport  Port=6
  pqrdot : Inport  Port=7
  Accels : Inport  Port=8
  abe : Inport  Port=9
  mass : Inport  Port=10
  EnvmData : Inport  Port=11
  Control : Inport  Port=12
  daohang : Inport  Port=13
  KFout : Inport  Port=14
  5 : Selector  InputPortWidth=3  IndexOptions=Index vector (dialog)  Indices=3  OutputSizes=1
  Airspeed : Sqrt  AlgorithmType=Newton-Raphson  SaturateOnIntegerOverflow=on
  Bus Creator : BusCreator  Inputs=20
  Bus Selector4 : BusSelector  OutputSignals=hground,g,To,Po
  Gain : Gain  Gain=-1
  Subsystem : Subsystem
  Sum : Sum  Inputs=+-|
  dot : Subsystem
  "nb & gb " : Subsystem
  Data : Outport
  wires:
  Euler/1 -> Subsystem/1(Ein)
  EnvmData/1 -> Bus Selector4/1
  Ve/1 -> dot/1(Vb), Bus Creator/1  "Ve"
  Xe/1 -> 5/1, Bus Creator/2  "Xe"
  5/1 -> Gain/1
  Gain/1 -> Bus Creator/3, Sum/1  "H"
  DCM/1 -> Bus Creator/6, "nb & gb "/1(DCM)  "DCM"
  Bus Selector4/1 -> Sum/2  "<hground>"
  Accels/1 -> Bus Creator/13, "nb & gb "/3(a)  "Accels"
  Bus Selector4/2 -> "nb & gb "/2(g)  "<g>"
  Sum/1 -> Bus Creator/4  "Hag"
  Subsystem/1(E) -> Bus Creator/5  "Euler"
  Vb/1 -> Bus Creator/7  "Vb"
  pqr/1 -> Bus Creator/8  "pqr"
  pqrdot/1 -> Bus Creator/9  "pqrdot"
  "nb & gb "/1(nb) -> Bus Creator/10  "nb"
  "nb & gb "/2(gb) -> Bus Creator/11  "gb"
  mass/1 -> Bus Creator/12  "mass"
  Bus Creator/1 -> Data/1
  abe/1 -> Bus Creator/14  "Accelsbe"
  dot/1(dot) -> Airspeed/1
  Airspeed/1 -> Bus Creator/15  "Va"
  Bus Selector4/3 -> Bus Creator/16  "<To>"
  Bus Selector4/4 -> Bus Creator/17  "<Po>"
  Control/1 -> Bus Creator/18  "control"
  daohang/1 -> Bus Creator/19  "daohang"
  KFout/1 -> Bus Creator/20  "KFout"

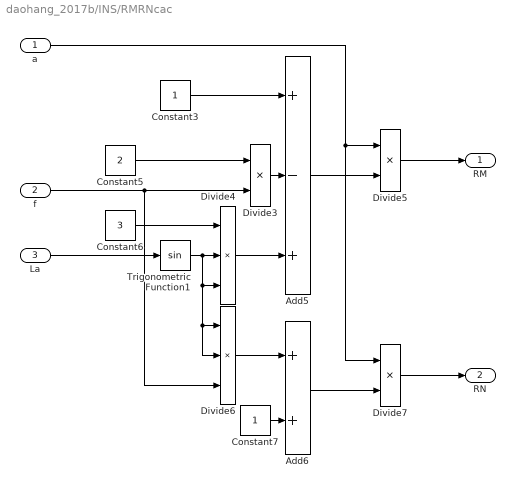
== system daohang_2017b/INS/RMRNcac ==
  a : Inport
  f : Inport  Port=2
  La : Inport  Port=3
  Add5 : Sum  Inputs=+-+
  Add6 : Sum
  Constant3 : Constant
  Constant5 : Constant  Value=2
  Constant6 : Constant  Value=3
  Constant7 : Constant
  Divide3 : Product  Inputs=**
  Divide4 : Product  Inputs=***
  Divide5 : Product  Inputs=**
  Divide6 : Product  Inputs=***
  Divide7 : Product  Inputs=**
  Trigonometric Function1 : Trigonometry
  RM : Outport
  RN : Outport  Port=2
  wires:
  Trigonometric Function1/1 -> Divide4/3, Divide6/1, Divide6/2, Divide4/2
  Divide6/1 -> Add6/1
  f/1 -> Divide6/3, Divide3/2
  Divide3/1 -> Add5/2
  Constant3/1 -> Add5/1
  Divide4/1 -> Add5/3
  Constant6/1 -> Divide4/1
  Constant7/1 -> Add6/2
  Add6/1 -> Divide7/2
  a/1 -> Divide7/1, Divide5/1
  Constant5/1 -> Divide3/1
  Add5/1 -> Divide5/2
  La/1 -> Trigonometric Function1/1
  Divide7/1 -> RN/1
  Divide5/1 -> RM/1

== system daohang_2017b/KF/Subsystem ==
  "NED " : Inport
  Demux1 : Demux  Outputs=3
  Gain3 : Gain  Gain=-1
  Mux1 : Mux  Inputs=3
  ENU : Outport
  wires:
  Gain3/1 -> Mux1/3
  Mux1/1 -> ENU/1
  Demux1/1 -> Mux1/2
  Demux1/2 -> Mux1/1
  "NED "/1 -> Demux1/1
  Demux1/3 -> Gain3/1

== system daohang_2017b/KF/Subsystem1 ==
  "NED " : Inport
  Demux1 : Demux  Outputs=3
  Gain3 : Gain  Gain=-1
  Mux1 : Mux  Inputs=3
  ENU : Outport
  wires:
  Gain3/1 -> Mux1/3
  Mux1/1 -> ENU/1
  Demux1/1 -> Mux1/2
  Demux1/2 -> Mux1/1
  "NED "/1 -> Demux1/1
  Demux1/3 -> Gain3/1

== system daohang_2017b/KF/Subsystem2 ==
  "ENU " : Inport
  Demux1 : Demux  Outputs=3
  Gain3 : Gain  Gain=-1
  Mux1 : Mux  Inputs=3
  NED : Outport
  wires:
  Gain3/1 -> Mux1/3
  Mux1/1 -> NED/1
  Demux1/1 -> Mux1/2
  Demux1/2 -> Mux1/1
  "ENU "/1 -> Demux1/1
  Demux1/3 -> Gain3/1

== system daohang_2017b/偏差/Subsystem ==
  raw signal : Inport
  Add3 : Sum  Inputs=+++
  Markov process : Subsystem
  Memory : Memory
  Random Number4 : RandomNumber  Variance=ini.H_Variance  Seed=51  SampleTime=0.01
  noise added : Outport
  wires:
  Add3/1 -> noise added/1
  Markov process/1(Markov noise) -> Add3/3
  Random Number4/1 -> Memory/1
  Memory/1 -> Add3/2
  raw signal/1 -> Add3/1

== system daohang_2017b/偏差/add noise ==
  raw signals : Inport
  Demux1 : Demux  Outputs=3
  Mux1 : Mux  Inputs=3
  Subsystem : Subsystem
  Subsystem1 : Subsystem
  Subsystem2 : Subsystem
  noise added signals : Outport
  wires:
  Demux1/3 -> Subsystem2/1(raw signal)
  Demux1/1 -> Subsystem/1(raw signal)
  Mux1/1 -> noise added signals/1
  Subsystem2/1(noise added) -> Mux1/3
  Subsystem/1(noise added) -> Mux1/1
  Demux1/2 -> Subsystem1/1(raw signal)
  Subsystem1/1(noise added) -> Mux1/2
  raw signals/1 -> Demux1/1

== system daohang_2017b/偏差/add noise1 ==
  raw signals : Inport
  Demux1 : Demux  Outputs=2
  Mux1 : Mux  Inputs=2
  Subsystem : Subsystem
  Subsystem1 : Subsystem
  noise added signals : Outport
  wires:
  Demux1/1 -> Subsystem/1(raw signal)
  Mux1/1 -> noise added signals/1
  Subsystem/1(noise added) -> Mux1/1
  Demux1/2 -> Subsystem1/1(raw signal)
  Subsystem1/1(noise added) -> Mux1/2
  raw signals/1 -> Demux1/1

== system daohang_2017b/偏差/add noise2 ==
  raw signals : Inport
  Demux1 : Demux  Outputs=3
  Mux1 : Mux  Inputs=3
  Subsystem : Subsystem
  Subsystem1 : Subsystem
  Subsystem2 : Subsystem
  noise added signals : Outport
  wires:
  Demux1/3 -> Subsystem2/1(raw signal)
  Demux1/1 -> Subsystem/1(raw signal)
  Mux1/1 -> noise added signals/1
  Subsystem2/1(noise added) -> Mux1/3
  Subsystem/1(noise added) -> Mux1/1
  Demux1/2 -> Subsystem1/1(raw signal)
  Subsystem1/1(noise added) -> Mux1/2
  raw signals/1 -> Demux1/1

== system daohang_2017b/偏差/add noise3 ==
  raw signals : Inport
  Demux1 : Demux  Outputs=3
  Mux1 : Mux  Inputs=3
  Subsystem : Subsystem
  Subsystem1 : Subsystem
  Subsystem2 : Subsystem
  noise added signals : Outport
  wires:
  Demux1/3 -> Subsystem2/1(raw signal)
  Demux1/1 -> Subsystem/1(raw signal)
  Mux1/1 -> noise added signals/1
  Subsystem2/1(noise added) -> Mux1/3
  Subsystem/1(noise added) -> Mux1/1
  Demux1/2 -> Subsystem1/1(raw signal)
  Subsystem1/1(noise added) -> Mux1/2
  raw signals/1 -> Demux1/1

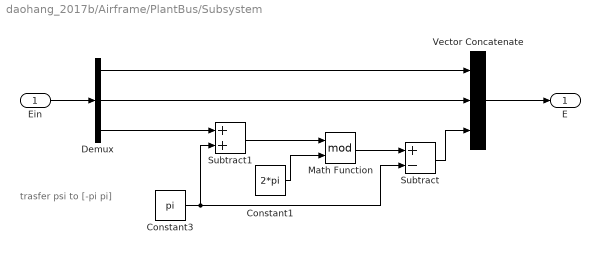
== system daohang_2017b/Airframe/PlantBus/Subsystem ==
  note: trasfer psi to [-pi pi]
  Ein : Inport
  Constant1 : Constant  Value=2*pi
  Constant3 : Constant  Value=pi
  Demux : Demux  Outputs=3
  Math Function : Math  Operator=mod  SaturateOnIntegerOverflow=on
  Subtract : Sum  Inputs=+-
  Subtract1 : Sum
  Vector Concatenate : Concatenate  NumInputs=3
  E : Outport
  wires:
  Constant1/1 -> Math Function/2
  Math Function/1 -> Subtract/1
  Subtract1/1 -> Math Function/1
  Constant3/1 -> Subtract1/2, Subtract/2
  Demux/3 -> Subtract1/1
  Subtract/1 -> Vector Concatenate/3
  Ein/1 -> Demux/1
  Demux/1 -> Vector Concatenate/1
  Demux/2 -> Vector Concatenate/2
  Vector Concatenate/1 -> E/1

== system daohang_2017b/Airframe/PlantBus/dot ==
  Vb : Inport
  Demux1 : Demux  Outputs=3
  Product : Product  RndMeth=Zero
  Product1 : Product  RndMeth=Zero
  Product2 : Product  RndMeth=Zero
  Sum : Sum  Inputs=+++
  dot : Outport
  wires:
  Product2/1 -> Sum/3
  Demux1/3 -> Product2/2, Product2/1
  Product/1 -> Sum/1
  Product1/1 -> Sum/2
  Sum/1 -> dot/1
  Vb/1 -> Demux1/1
  Demux1/1 -> Product/2, Product/1
  Demux1/2 -> Product1/1, Product1/2

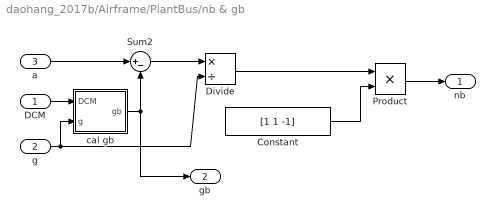
== system daohang_2017b/Airframe/PlantBus/nb & gb  ==
  DCM : Inport
  g : Inport  Port=2
  a : Inport  Port=3
  Constant : Constant  Value=[1 1 -1]
  Divide : Product  Inputs=*/
  Product : Product  RndMeth=Zero
  Sum2 : Sum  Inputs=|+-
  cal gb : Subsystem
  nb : Outport
  gb : Outport  Port=2
  wires:
  Product/1 -> nb/1
  Constant/1 -> Product/2
  Divide/1 -> Product/1
  g/1 -> Divide/2, cal gb/2(g)
  a/1 -> Sum2/1
  Sum2/1 -> Divide/1
  cal gb/1(gb) -> Sum2/2, gb/1
  DCM/1 -> cal gb/1(DCM)

== system daohang_2017b/偏差/Subsystem/Markov process ==
  Add12 : Sum
  Gain : Gain  Gain=-1/ini.M_H_T
  Integrator : Integrator
  Memory11 : Memory
  Random Number13 : RandomNumber  Variance=ini.M_H_Variance  Seed=52  SampleTime=0.01
  Markov noise : Outport
  wires:
  Memory11/1 -> Gain/1
  Gain/1 -> Integrator/1
  Add12/1 -> Markov noise/1, Memory11/1
  Integrator/1 -> Add12/1
  Random Number13/1 -> Add12/2

== system daohang_2017b/偏差/add noise/Subsystem ==
  raw signal : Inport
  Add3 : Sum  Inputs=+++
  Markov process : Subsystem
  Memory : Memory
  Random Number4 : RandomNumber  Variance=(ini.omega_Variance/3600/180*pi)^2  Seed=11  SampleTime=0.01
  noise added : Outport
  wires:
  Add3/1 -> noise added/1
  Markov process/1(Markov noise) -> Add3/3
  Random Number4/1 -> Memory/1
  Memory/1 -> Add3/2
  raw signal/1 -> Add3/1

== system daohang_2017b/偏差/add noise/Subsystem1 ==
  raw signal : Inport
  Add3 : Sum  Inputs=+++
  Markov process : Subsystem
  Memory : Memory
  Random Number4 : RandomNumber  Variance=(ini.omega_Variance/3600/180*pi)^2  Seed=13  SampleTime=0.01
  noise added : Outport
  wires:
  Add3/1 -> noise added/1
  Markov process/1(Markov noise) -> Add3/3
  Random Number4/1 -> Memory/1
  Memory/1 -> Add3/2
  raw signal/1 -> Add3/1

== system daohang_2017b/偏差/add noise/Subsystem2 ==
  raw signal : Inport
  Add3 : Sum  Inputs=+++
  Markov process : Subsystem
  Memory : Memory
  Random Number4 : RandomNumber  Variance=(ini.omega_Variance/3600/180*pi)^2  Seed=15  SampleTime=0.01
  noise added : Outport
  wires:
  Add3/1 -> noise added/1
  Markov process/1(Markov noise) -> Add3/3
  Random Number4/1 -> Memory/1
  Memory/1 -> Add3/2
  raw signal/1 -> Add3/1

== system daohang_2017b/偏差/add noise1/Subsystem ==
  raw signal : Inport
  Add3 : Sum  Inputs=+++
  Markov process : Subsystem
  Memory : Memory
  Random Number4 : RandomNumber  Variance=ini.GPS_Variance  Seed=1  SampleTime=0.01
  noise added : Outport
  wires:
  Add3/1 -> noise added/1
  Markov process/1(Markov noise) -> Add3/3
  Random Number4/1 -> Memory/1
  Memory/1 -> Add3/2
  raw signal/1 -> Add3/1

== system daohang_2017b/偏差/add noise1/Subsystem1 ==
  raw signal : Inport
  Add3 : Sum  Inputs=+++
  Markov process : Subsystem
  Memory : Memory
  Random Number4 : RandomNumber  Variance=ini.GPS_Variance  Seed=3  SampleTime=0.01
  noise added : Outport
  wires:
  Add3/1 -> noise added/1
  Markov process/1(Markov noise) -> Add3/3
  Random Number4/1 -> Memory/1
  Memory/1 -> Add3/2
  raw signal/1 -> Add3/1

== system daohang_2017b/偏差/add noise2/Subsystem ==
  raw signal : Inport
  Add3 : Sum  Inputs=+++
  Markov process : Subsystem
  Memory : Memory
  Random Number4 : RandomNumber  Variance=(ini.a_Variance/3600)^2  Seed=21  SampleTime=0.01
  noise added : Outport
  wires:
  Add3/1 -> noise added/1
  Markov process/1(Markov noise) -> Add3/3
  Random Number4/1 -> Memory/1
  Memory/1 -> Add3/2
  raw signal/1 -> Add3/1

== system daohang_2017b/偏差/add noise2/Subsystem1 ==
  raw signal : Inport
  Add3 : Sum  Inputs=+++
  Markov process : Subsystem
  Memory : Memory
  Random Number4 : RandomNumber  Variance=(ini.a_Variance/3600)^2  Seed=23  SampleTime=0.01
  noise added : Outport
  wires:
  Add3/1 -> noise added/1
  Markov process/1(Markov noise) -> Add3/3
  Random Number4/1 -> Memory/1
  Memory/1 -> Add3/2
  raw signal/1 -> Add3/1

== system daohang_2017b/偏差/add noise2/Subsystem2 ==
  raw signal : Inport
  Add3 : Sum  Inputs=+++
  Markov process : Subsystem
  Memory : Memory
  Random Number4 : RandomNumber  Variance=(ini.a_Variance/3600)^2  Seed=26  SampleTime=0.01
  noise added : Outport
  wires:
  Add3/1 -> noise added/1
  Markov process/1(Markov noise) -> Add3/3
  Random Number4/1 -> Memory/1
  Memory/1 -> Add3/2
  raw signal/1 -> Add3/1

== system daohang_2017b/偏差/add noise3/Subsystem ==
  raw signal : Inport
  Add3 : Sum  Inputs=+++
  Markov process : Subsystem
  Memory : Memory
  Random Number4 : RandomNumber  Variance=ini.V_Variance  Seed=31  SampleTime=0.01
  noise added : Outport
  wires:
  Add3/1 -> noise added/1
  Markov process/1(Markov noise) -> Add3/3
  Random Number4/1 -> Memory/1
  Memory/1 -> Add3/2
  raw signal/1 -> Add3/1

== system daohang_2017b/偏差/add noise3/Subsystem1 ==
  raw signal : Inport
  Add3 : Sum  Inputs=+++
  Markov process : Subsystem
  Memory : Memory
  Random Number4 : RandomNumber  Variance=ini.V_Variance  Seed=43  SampleTime=0.01
  noise added : Outport
  wires:
  Add3/1 -> noise added/1
  Markov process/1(Markov noise) -> Add3/3
  Random Number4/1 -> Memory/1
  Memory/1 -> Add3/2
  raw signal/1 -> Add3/1

== system daohang_2017b/偏差/add noise3/Subsystem2 ==
  raw signal : Inport
  Add3 : Sum  Inputs=+++
  Markov process : Subsystem
  Memory : Memory
  Random Number4 : RandomNumber  Variance=ini.V_Variance  Seed=45  SampleTime=0.01
  noise added : Outport
  wires:
  Add3/1 -> noise added/1
  Markov process/1(Markov noise) -> Add3/3
  Random Number4/1 -> Memory/1
  Memory/1 -> Add3/2
  raw signal/1 -> Add3/1

== system daohang_2017b/Airframe/PlantBus/nb & gb /cal gb ==
  DCM : Inport
  g : Inport  Port=2
  Constant2 : Constant  Value=0
  Mux : Mux  Inputs=3
  To Body Axes : Product  Multiplication=Matrix(*)  SaturateOnIntegerOverflow=on  InputSameDT=on  OutDataTypeStr=Inherit: Same as first input
  gb : Outport
  wires:
  Mux/1 -> To Body Axes/2
  Constant2/1 -> Mux/1, Mux/2
  DCM/1 -> To Body Axes/1
  To Body Axes/1 -> gb/1
  g/1 -> Mux/3

== system daohang_2017b/偏差/add noise/Subsystem/Markov process ==
  Add12 : Sum
  Gain : Gain  Gain=-1/ini.M_omega_T
  Integrator : Integrator
  Memory11 : Memory
  Random Number13 : RandomNumber  Variance=(ini.M_omega_Variance/3600/180*pi)^2  Seed=12  SampleTime=0.01
  Markov noise : Outport
  wires:
  Memory11/1 -> Gain/1
  Gain/1 -> Integrator/1
  Add12/1 -> Markov noise/1, Memory11/1
  Integrator/1 -> Add12/1
  Random Number13/1 -> Add12/2

== system daohang_2017b/偏差/add noise/Subsystem1/Markov process ==
  Add12 : Sum
  Gain : Gain  Gain=-1/ini.M_omega_T
  Integrator : Integrator
  Memory11 : Memory
  Random Number13 : RandomNumber  Variance=(ini.M_omega_Variance/3600/180*pi)^2  Seed=14  SampleTime=0.01
  Markov noise : Outport
  wires:
  Memory11/1 -> Gain/1
  Gain/1 -> Integrator/1
  Add12/1 -> Markov noise/1, Memory11/1
  Integrator/1 -> Add12/1
  Random Number13/1 -> Add12/2

== system daohang_2017b/偏差/add noise/Subsystem2/Markov process ==
  Add12 : Sum
  Gain : Gain  Gain=-1/ini.M_omega_T
  Integrator : Integrator
  Memory11 : Memory
  Random Number13 : RandomNumber  Variance=(ini.M_omega_Variance/3600/180*pi)^2  Seed=16  SampleTime=0.01
  Markov noise : Outport
  wires:
  Memory11/1 -> Gain/1
  Gain/1 -> Integrator/1
  Add12/1 -> Markov noise/1, Memory11/1
  Integrator/1 -> Add12/1
  Random Number13/1 -> Add12/2

== system daohang_2017b/偏差/add noise1/Subsystem/Markov process ==
  Add12 : Sum
  Gain : Gain  Gain=-1/ini.M_GPS_T
  Integrator : Integrator
  Memory11 : Memory
  Random Number13 : RandomNumber  Variance=ini.M_GPS_Variance  Seed=2  SampleTime=0.01
  Markov noise : Outport
  wires:
  Memory11/1 -> Gain/1
  Gain/1 -> Integrator/1
  Add12/1 -> Markov noise/1, Memory11/1
  Integrator/1 -> Add12/1
  Random Number13/1 -> Add12/2

== system daohang_2017b/偏差/add noise1/Subsystem1/Markov process ==
  Add12 : Sum
  Gain : Gain  Gain=-1/ini.M_GPS_T
  Integrator : Integrator
  Memory11 : Memory
  Random Number13 : RandomNumber  Variance=ini.M_GPS_Variance  Seed=4  SampleTime=0.01
  Markov noise : Outport
  wires:
  Memory11/1 -> Gain/1
  Gain/1 -> Integrator/1
  Add12/1 -> Markov noise/1, Memory11/1
  Integrator/1 -> Add12/1
  Random Number13/1 -> Add12/2

== system daohang_2017b/偏差/add noise2/Subsystem/Markov process ==
  Add12 : Sum
  Gain : Gain  Gain=-1/ini.M_a_T
  Integrator : Integrator
  Memory11 : Memory
  Random Number13 : RandomNumber  Variance=(ini.M_a_Variance/3600)^2  Seed=22  SampleTime=0.01
  Markov noise : Outport
  wires:
  Memory11/1 -> Gain/1
  Gain/1 -> Integrator/1
  Add12/1 -> Markov noise/1, Memory11/1
  Integrator/1 -> Add12/1
  Random Number13/1 -> Add12/2

== system daohang_2017b/偏差/add noise2/Subsystem1/Markov process ==
  Add12 : Sum
  Gain : Gain  Gain=-1/ini.M_a_T
  Integrator : Integrator
  Memory11 : Memory
  Random Number13 : RandomNumber  Variance=(ini.M_a_Variance/3600)^2  Seed=24  SampleTime=0.01
  Markov noise : Outport
  wires:
  Memory11/1 -> Gain/1
  Gain/1 -> Integrator/1
  Add12/1 -> Markov noise/1, Memory11/1
  Integrator/1 -> Add12/1
  Random Number13/1 -> Add12/2

== system daohang_2017b/偏差/add noise2/Subsystem2/Markov process ==
  Add12 : Sum
  Gain : Gain  Gain=-1/ini.M_a_T
  Integrator : Integrator
  Memory11 : Memory
  Random Number13 : RandomNumber  Variance=(ini.M_a_Variance/3600)^2  Seed=27  SampleTime=0.01
  Markov noise : Outport
  wires:
  Memory11/1 -> Gain/1
  Gain/1 -> Integrator/1
  Add12/1 -> Markov noise/1, Memory11/1
  Integrator/1 -> Add12/1
  Random Number13/1 -> Add12/2

== system daohang_2017b/偏差/add noise3/Subsystem/Markov process ==
  Add12 : Sum
  Gain : Gain  Gain=-1/ini.M_V_T
  Integrator : Integrator
  Memory11 : Memory
  Random Number13 : RandomNumber  Variance=ini.M_V_Variance  Seed=42  SampleTime=0.01
  Markov noise : Outport
  wires:
  Memory11/1 -> Gain/1
  Gain/1 -> Integrator/1
  Add12/1 -> Markov noise/1, Memory11/1
  Integrator/1 -> Add12/1
  Random Number13/1 -> Add12/2

== system daohang_2017b/偏差/add noise3/Subsystem1/Markov process ==
  Add12 : Sum
  Gain : Gain  Gain=-1/ini.M_V_T
  Integrator : Integrator
  Memory11 : Memory
  Random Number13 : RandomNumber  Variance=ini.M_V_Variance  Seed=44  SampleTime=0.01
  Markov noise : Outport
  wires:
  Memory11/1 -> Gain/1
  Gain/1 -> Integrator/1
  Add12/1 -> Markov noise/1, Memory11/1
  Integrator/1 -> Add12/1
  Random Number13/1 -> Add12/2
